simulink model "actuator_ident"  (R2018b)
settings: Solver=ode4  StartTime=0.0  StopTime=1000  FixedStep=0.01  RelTol=1e-3
settings Model: Creator=ge34qer  LastModifiedBy=ge34qer

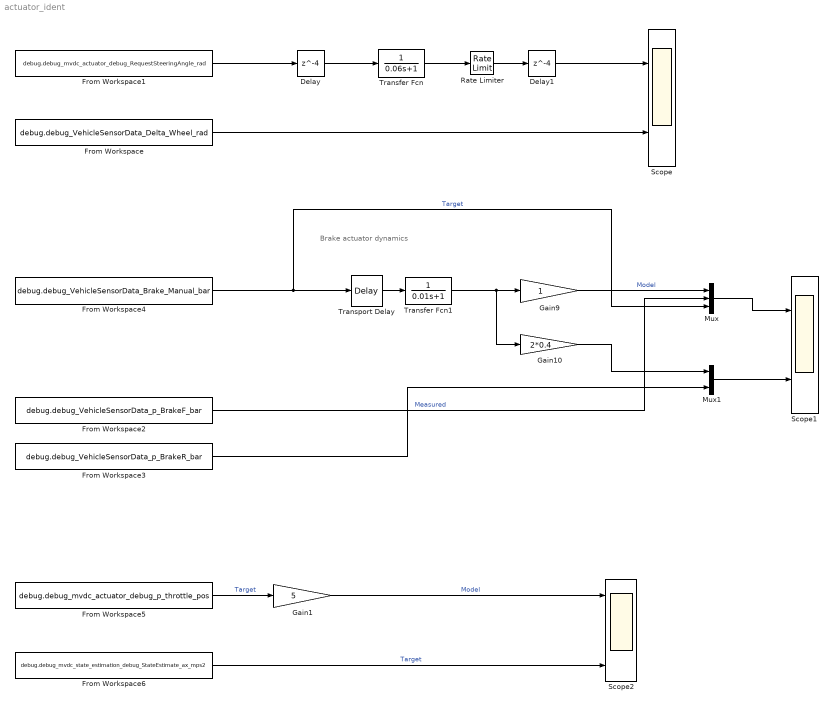
== system actuator_ident ==
  note: Brake actuator dynamics
  Delay : Delay  DelayLength=4
  Delay1 : Delay  DelayLength=4
  From Workspace : FromWorkspace  VariableName=debug.debug_VehicleSensorData_Delta_Wheel_rad  SampleTime=0
  From Workspace1 : FromWorkspace  VariableName=debug.debug_mvdc_actuator_debug_RequestSteeringAngle_rad  SampleTime=0
  From Workspace2 : FromWorkspace  VariableName=debug.debug_VehicleSensorData_p_BrakeF_bar  SampleTime=0
  From Workspace3 : FromWorkspace  VariableName=debug.debug_VehicleSensorData_p_BrakeR_bar  SampleTime=0
  From Workspace4 : FromWorkspace  VariableName=debug.debug_VehicleSensorData_Brake_Manual_bar  SampleTime=0
  From Workspace5 : FromWorkspace  VariableName=debug.debug_mvdc_actuator_debug_p_throttle_pos  SampleTime=0
  From Workspace6 : FromWorkspace  VariableName=debug.debug_mvdc_state_estimation_debug_StateEstimate_ax_mps2  SampleTime=0
  Gain1 : Gain  Gain=5
  Gain10 : Gain  Gain=2*0.4
  Gain9 : Gain
  Mux : Mux  Inputs=3
  Mux1 : Mux  Inputs=2
  Rate Limiter : RateLimiter  RisingSlewLimit=6.28/19.5  FallingSlewLimit=-6.28/19.5  SampleTimeMode=inherited
  Scope : Scope  NumInputPorts=2
  Scope1 : Scope  NumInputPorts=2
  Scope2 : Scope  NumInputPorts=3
  Transfer Fcn : TransferFcn  Denominator=[0.06 1]
  Transfer Fcn1 : TransferFcn  Denominator=[0.01 1]
  Transport Delay : TransportDelay  DelayTime=0.02
  wires:
  From Workspace1/1 -> Delay/1
  From Workspace/1 -> Scope/2
  Delay/1 -> Transfer Fcn/1
  Transfer Fcn/1 -> Rate Limiter/1
  Delay1/1 -> Scope/1
  Rate Limiter/1 -> Delay1/1
  Gain10/1 -> Mux1/1
  Gain9/1 -> Mux/1  "Model"
  Transfer Fcn1/1 -> Gain10/1, Gain9/1
  Transport Delay/1 -> Transfer Fcn1/1
  Mux/1 -> Scope1/1
  From Workspace2/1 -> Mux/2  "Measured"
  Mux1/1 -> Scope1/2
  From Workspace3/1 -> Mux1/2
  From Workspace4/1 -> Mux/3, Transport Delay/1  "Target"
  From Workspace5/1 -> Gain1/1  "Target"
  Gain1/1 -> Scope2/1  "Model"
  From Workspace6/1 -> Scope2/3  "Target"
